simulink model "example_msg_attitude"  (R2017a)
settings: Solver=FixedStepAuto  StartTime=0.0  StopTime=10.0  FixedStep=0.01  RelTol=1e-3
libraries: dspnetwork x2, aerolibanimutils x1
settings Model: Creator=Admin  LastModifiedBy=Admin

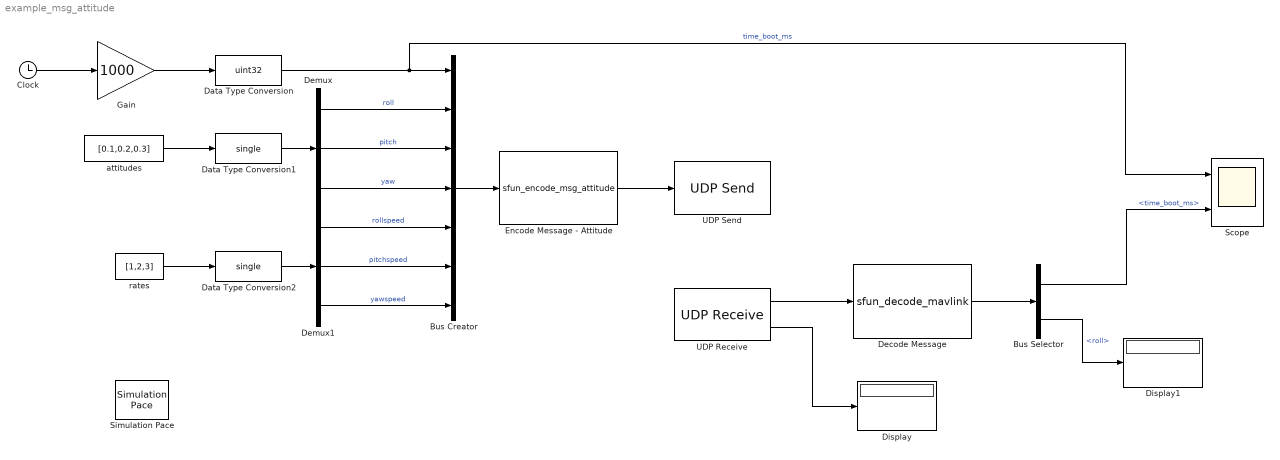
== system example_msg_attitude ==
  Bus Creator : BusCreator  Inputs=7  OutDataTypeStr=Bus: mavlink_attitude_t
  Bus Selector : BusSelector  OutputSignals=time_boot_ms,roll
  Clock : Clock
  Data Type Conversion : DataTypeConversion  OutDataTypeStr=uint32
  Data Type Conversion1 : DataTypeConversion  OutDataTypeStr=single
  Data Type Conversion2 : DataTypeConversion  OutDataTypeStr=single
  Decode Message : S-Function  FunctionName=sfun_decode_mavlink  SFunctionDeploymentMode=off  EnableBusSupport=off
  Demux : Demux  Outputs=3
  Demux1 : Demux  Outputs=3
  Display : Display
  Display1 : Display
  Encode Message - Attitude : S-Function  FunctionName=sfun_encode_msg_attitude  SFunctionDeploymentMode=off  EnableBusSupport=off
  Gain : Gain  Gain=1000
  Scope : Scope  NumInputPorts=2
  Simulation Pace : aerolibanimutils/Simulation Pace  SimulationPace=1  SleepMode=MATLAB Thread  OutputPaceError=off  SampleTime=0.01
  UDP Receive : dspnetwork/UDP Receive  localURL='0.0.0.0'  localPort=25000  remoteURL='0.0.0.0'  remotePort=-1  recvBufferSize=8192  dims=263  signalDatatype=uint8  isVarSize=off  showBlockingTime=on  blockingTime=0  sampletime=0.01  blockPlatform=HOST
  UDP Send : dspnetwork/UDP Send  remoteURL='255.255.255.255'  remotePort=25000  localURL='0.0.0.0'  localPortSource=Automatically determine  localPort=-1  sampletime=-1  blockPlatform=HOST  separateLengthPort=0
  attitudes : Constant  Value=[0.1,0.2,0.3]
  rates : Constant  Value=[1,2,3]
  wires:
  Encode Message - Attitude/1 -> UDP Send/1
  Bus Creator/1 -> Encode Message - Attitude/1
  Data Type Conversion/1 -> Scope/1, Bus Creator/1  "time_boot_ms"
  Clock/1 -> Gain/1
  Demux/1 -> Bus Creator/2  "roll"
  Demux/2 -> Bus Creator/3  "pitch"
  Demux/3 -> Bus Creator/4  "yaw"
  Demux1/1 -> Bus Creator/5  "rollspeed"
  Demux1/2 -> Bus Creator/6  "pitchspeed"
  Demux1/3 -> Bus Creator/7  "yawspeed"
  Data Type Conversion1/1 -> Demux/1
  Data Type Conversion2/1 -> Demux1/1
  attitudes/1 -> Data Type Conversion1/1
  rates/1 -> Data Type Conversion2/1
  UDP Receive/1 -> Decode Message/1
  Decode Message/1 -> Bus Selector/1
  Bus Selector/1 -> Scope/2  "<time_boot_ms>"
  UDP Receive/2 -> Display/1
  Gain/1 -> Data Type Conversion/1
  Bus Selector/2 -> Display1/1  "<roll>"
